simulink model "lqr_quad"  (R2023a)
settings: Solver=VariableStepAuto  StartTime=0.0  StopTime=inf  RelTol=1e-3
undefined symbols (not defined in the file): A_sys, B_sys, C_sys, D_sys
libraries: vrlib x1
settings Model: Creator=sait karadeniz  LastModifiedBy=sait karadeniz
settings DataIOCC: ReturnWorkspaceOutputs=off

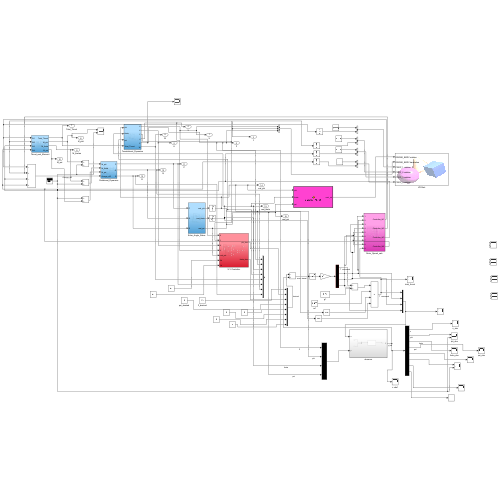
[thumbnail: Simulink's stored preview of the top-level diagram]
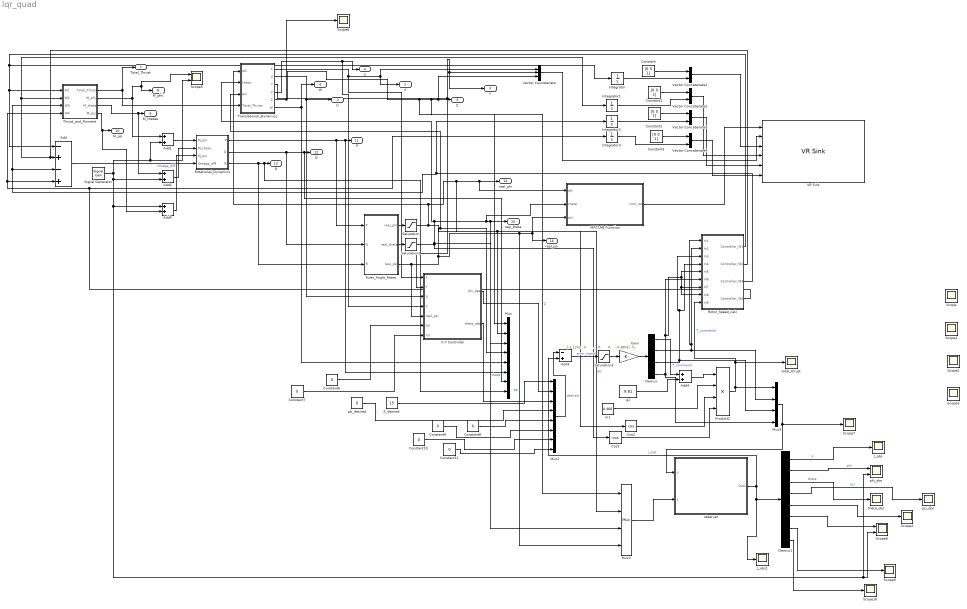
== system lqr_quad ==
  Add : Sum  Inputs=-+-+
  Add{1..2,4..5} (4 alike) : Sum
  Add3 : Sum  Inputs=-+
  Constant{,1..3} (4 alike) : Constant  Value=[0 0 1]  OutMax=[3]
  Constant{6..11} (6 alike) : Constant  Value=0
  Cos2 : Trigonometry  Operator=cos
  Cos3 : Trigonometry  Operator=cos
  Demux : Demux
  Demux1 : Demux  Outputs=8
  Euler_Angle_Rates : Subsystem
  Gain : Gain  Gain=|  Multiplication=Matrix(K*u)
      | [-1.1243,  0,       0,       0,     -0.9940,  0,       0,       0;
      |   0,      -1.6555,  0,       0,      0,      -0.0231,  0,       0;
      |   0,       0,      -2.0992,  0,      0,       0,     -0.1455,  0;
      |   0,       0,       0,     -1.1305,  0,       0,       0,     -0.3803]
  Integrator{,1..3} (4 alike) : Integrator
  MATLAB Function : MATLAB Function  TreatAsAtomicUnit=on
  Mux : Mux  Inputs=8
  Mux1 : Mux  Inputs=8
  Mux2 : Mux
  Mux3 : Mux
  Product2 : Product  Inputs=4
  Rotational_Dynamics : Subsystem
  Rotor_Speed_calc : Subsystem
  Saturation : Saturate  UpperLimit=pi/2  LowerLimit=-pi/2
  Saturation1 : Saturate  UpperLimit=pi/2  LowerLimit=-pi/2
  Saturation3 : Saturate  UpperLimit=500  LowerLimit=-5
  Scope{,1..3,5,8} (6 alike) : Scope  NumInputPorts=2
  Scope{4,6..7,9..10} (5 alike) : Scope
  Signal Generator : SignalGenerator  Amplitude=0.002  Frequency=3  Units=rad/sec
  Thrust_and_Moment : Subsystem
  Translational_Dynamics : Subsystem
  VR Sink : vrlib/VR Sink  InstantiateOnLoad=on  SampleTime=0.1  ViewEnable=on  RemoteChange=off  RemoteView=off  FieldsWritten=DRONE_BODY.rotation.4.1.1.double#DRONE_BODY.translation.3.1.1.double#PROP_1.rotation.4.1.1.double#PROP_2.rotation.4.1.1.double#PROP_3.rotation.4.1.1.double#PROP_4.rotation.4.1.1.double  WorldFileName=C:\Documents\quadcopter.wrl  WorldDescription=Quadcopter World  AutoView=on  VideoDimensions=[]  AllowVariableSize=off  FigureProperties="{'Position', 'Name', 'Viewpoint', 'CameraBound', 'CameraDirection', 'CameraPosition', 'CameraUpVector', 'ZoomFactor', 'Antialiasing', 'Headlight', 'Lighting', 'NavPanel', 'Sound', 'StatusBar', 'Stereo3D', 'Stereo3DCameraOffset', 'Stereo3DHIT', 'ToolBar', 'Textures', 'Transparency', 'Triad', 'Wireframe', 'NavZones', 'NavMode', 'NavSpeed', 'CaptureFileFormat', 'CaptureFileName', 'Record2DCompressMethod', 'Record2DCompressQuality', 'Record2D', 'Record2DFileName', 'Record2DFPS'; [8.8180000000000007e+02   1.8300000000000000e+02   5.7600000000000000e+02   5.0760000000000002e+02], 'Quadcopter World', 'Front View', 'on', [-6.4578595001307049e-01  -1.2433086949529201e-01  -7.5332751287603050e-01], [1.2901758596078691e+01   1.9679088050098620e+01   3.4424497589942021e+01], [-3.6247815328599153e-01  -8.1845083703478472e-01   4.4581141276029251e-01], [1.0000000000000000e+00], 'on', 'on', 'on', 'halfbar', 'on', 'on', 'off', [1.0000000149011612e-01], [0.0000000000000000e+00], 'on', 'on', 'on', 'none', 'off', 'off', 'walk', 'normal', 'tif', '%f_anim_%n.tif', 'auto', [7.5000000000000000e+01], 'off', '%f_anim_%n.avi', 'auto'}"
  Vector Concatenate : Concatenate  NumInputs=3
  Vector Concatenate{1..4} (4 alike) : Concatenate
  X-Y Controller : Subsystem
  Z_desired : Constant  Value=15
  g1 : Constant  Value=9.81
  m1 : Constant  Value=0.468
  observer : Subsystem
  phi_obs : Scope  NumInputPorts=2
  psi_desired : Constant  Value=0
  psi_obs : Scope
  theta_obs : Scope
  total_thrust : Scope
  z_obs : Scope
  z_obs1 : Scope
  X : Outport
  U : Outport  Port=2
  Y : Outport  Port=3
  V : Outport  Port=4
  Z : Outport  Port=5
  W : Outport  Port=6
  Total_Thrust : Outport  Port=7
  M_phii : Outport  Port=8
  M_thetaa : Outport  Port=9
  M_psi : Outport  Port=10
  P : Outport  Port=11
  Q : Outport  Port=12
  R : Outport  Port=13
  real_phi : Outport  Port=14
  real_theta : Outport  Port=15
  real_psi : Outport  Port=16
  wires:
  X-Y Controller/2(theta_des) -> Mux1/3
  Translational_Dynamics/5(Z) -> Scope6/1, Mux2/1, Z/1, Vector Concatenate/3, Mux/1  "Z"
  Z_desired/1 -> Mux1/1
  X-Y Controller/1(phi_des) -> Mux1/2
  Add1/1 -> Rotational_Dynamics/1(M_phi)
  Signal Generator/1 -> Add2/2, Add5/1, phi_obs/2, Scope8/2, Scope5/2, Add1/2
  Integrator3/1 -> Vector Concatenate4/2
  Constant7/1 -> X-Y Controller/7(Yd)
  Euler_Angle_Rates/2(real_theta) -> Saturation1/1
  Constant2/1 -> Vector Concatenate3/1
  Rotor_Speed_calc/1(Controller_W1) -> Add/1, Thrust_and_Moment/1(W1), Integrator/1
  MATLAB Function/1(vrml_rot) -> VR Sink/1
  Rotational_Dynamics/2(Q) -> Euler_Angle_Rates/2(Q), Mux/7, Q/1
  Integrator2/1 -> Vector Concatenate3/2
  Thrust_and_Moment/3(M_theta) -> Add2/1, M_thetaa/1
  Rotor_Speed_calc/2(Controller_W2) -> Integrator1/1, Thrust_and_Moment/2(W2), Add/2
  Translational_Dynamics/1(X) -> Vector Concatenate/1, X/1, X-Y Controller/1(X)
  Vector Concatenate3/1 -> VR Sink/5
  Vector Concatenate2/1 -> VR Sink/4
  Constant3/1 -> Vector Concatenate4/1
  Integrator1/1 -> Vector Concatenate2/2
  Rotor_Speed_calc/4(Controller_W4) -> Thrust_and_Moment/4(W4), Add/4, Integrator3/1
  Vector Concatenate1/1 -> VR Sink/3
  psi_desired/1 -> Mux1/4
  Add/1 -> Rotational_Dynamics/4(Omega_diff)  "Omega_diff"
  Constant1/1 -> Vector Concatenate2/1
  Translational_Dynamics/3(Y) -> Y/1, Vector Concatenate/2, X-Y Controller/2(Y)
  Integrator/1 -> Vector Concatenate1/2
  Vector Concatenate4/1 -> VR Sink/6
  Rotor_Speed_calc/3(Controller_W3) -> Thrust_and_Moment/3(W3), Add/3, Integrator2/1
  Constant6/1 -> X-Y Controller/6(Xd)
  Rotational_Dynamics/3(R) -> Euler_Angle_Rates/3(R), Mux/8, R/1
  Thrust_and_Moment/4(M_psi) -> Add5/2, M_psi/1
  Thrust_and_Moment/2(M_phi) -> M_phii/1, Scope5/1, Add1/1
  Translational_Dynamics/4(V) -> V/1, X-Y Controller/4(V)
  Vector Concatenate/1 -> VR Sink/2
  Translational_Dynamics/6(W) -> W/1, Mux/5
  Translational_Dynamics/2(U) -> U/1, X-Y Controller/3(U)
  Constant/1 -> Vector Concatenate1/1
  Euler_Angle_Rates/1(real_phi) -> Saturation/1
  Thrust_and_Moment/1(Total_Thrust) -> Total_Thrust/1, Translational_Dynamics/4(Total_Thrust)
  Euler_Angle_Rates/3(real_psi) -> Mux/4, Translational_Dynamics/3(psi), Mux2/4, MATLAB Function/3(psi), real_psi/1, X-Y Controller/5(real_psi)  "psi"
  Rotational_Dynamics/1(P) -> Mux/6, P/1, Euler_Angle_Rates/1(P)
  Constant8/1 -> Mux1/5
  Constant9/1 -> Mux1/6
  Constant10/1 -> Mux1/7
  Constant11/1 -> Mux1/8
  Mux1/1 -> Add3/1  "desired"
  Gain/1 -> Demux/1
  Demux/2 -> Mux3/2, Rotor_Speed_calc/1(In1), Rotor_Speed_calc/2(In2)
  Demux/3 -> Rotor_Speed_calc/4(In4), Rotor_Speed_calc/3(In3), Mux3/3
  Demux/4 -> Mux3/4, Rotor_Speed_calc/5(In5), Rotor_Speed_calc/8(In8), Rotor_Speed_calc/7(In7), Rotor_Speed_calc/6(In6)
  Saturation/1 -> Cos2/1, Mux/2, Translational_Dynamics/1(phi), Mux2/2, MATLAB Function/1(phi), real_phi/1  "phi"
  Saturation1/1 -> Cos3/1, Translational_Dynamics/2(theta), Mux2/3, real_theta/1, MATLAB Function/2(theta), Mux/3  "theta"
  g1/1 -> Add4/2
  Cos3/1 -> Product2/4
  m1/1 -> Product2/2
  Product2/1 -> total_thrust/1, Rotor_Speed_calc/9(In9), Mux3/1  "T_command"
  Add4/1 -> Product2/1
  Cos2/1 -> Product2/3
  Demux/1 -> Add4/1  "T_command"
  Add3/1 -> Saturation3/1  "error_signal"
  Saturation3/1 -> Gain/1
  Mux2/1 -> observer/2(y)
  observer/1(Out1) -> Add3/2, z_obs1/1, Demux1/1  "x_hat"
  Demux1/1 -> z_obs/1  "z"
  Demux1/2 -> phi_obs/1  "phi"
  Demux1/3 -> theta_obs/1  "theta"
  Demux1/4 -> psi_obs/1  "psi"
  Mux3/1 -> observer/1(u), Scope7/1
  Demux1/5 -> Scope4/1
  Demux1/6 -> Scope8/1
  Demux1/7 -> Scope9/1
  Demux1/8 -> Scope10/1
  Add2/1 -> Rotational_Dynamics/2(M_theta)
  Add5/1 -> Rotational_Dynamics/3(M_psi)

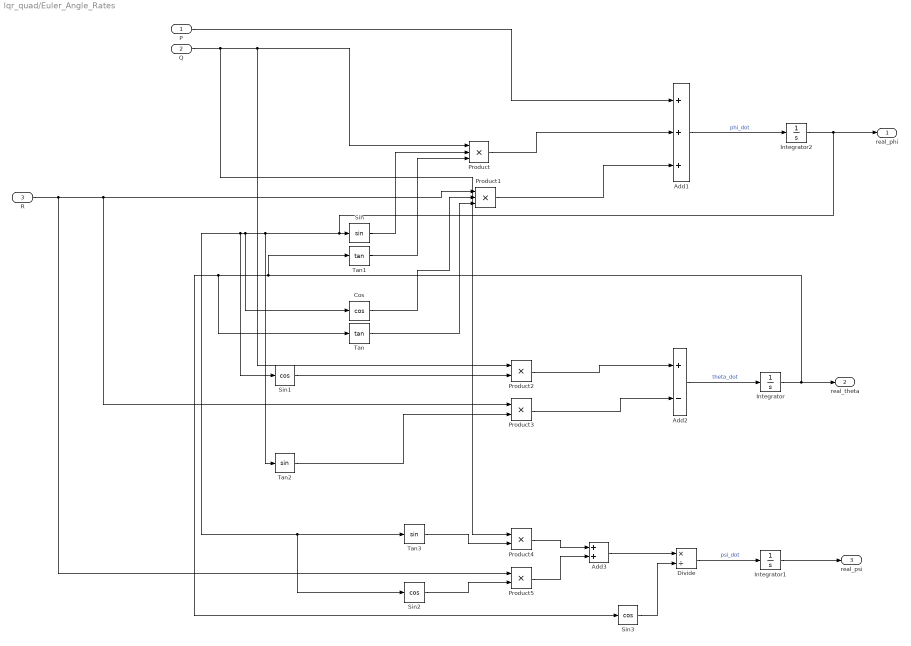
== system lqr_quad/Euler_Angle_Rates ==
  P : Inport
  Q : Inport  Port=2
  R : Inport  Port=3
  Add1 : Sum  Inputs=+++
  Add2 : Sum  Inputs=+-
  Add3 : Sum
  Cos : Trigonometry  Operator=cos
  Divide : Product  Inputs=*/
  Integrator : Integrator
  Integrator1 : Integrator
  Integrator2 : Integrator
  Product : Product  Inputs=3
  Product1 : Product  Inputs=3
  Product{2..5} (4 alike) : Product
  Sin : Trigonometry
  Sin1 : Trigonometry  Operator=cos
  Sin2 : Trigonometry  Operator=cos
  Sin3 : Trigonometry  Operator=cos
  Tan : Trigonometry  Operator=tan
  Tan1 : Trigonometry  Operator=tan
  Tan2 : Trigonometry
  Tan3 : Trigonometry
  real_phi : Outport
  real_theta : Outport  Port=2
  real_psi : Outport  Port=3
  wires:
  Tan1/1 -> Product/3
  Integrator2/1 -> real_phi/1, Sin2/1, Tan3/1, Sin1/1, Cos/1, Tan2/1, Sin/1
  Add1/1 -> Integrator2/1  "phi_dot"
  Divide/1 -> Integrator1/1  "psi_dot"
  Product3/1 -> Add2/2
  Integrator/1 -> real_theta/1, Sin3/1, Tan/1, Tan1/1
  Product1/1 -> Add1/3
  Tan3/1 -> Product4/2
  Sin2/1 -> Product5/2
  Tan2/1 -> Product3/2
  Integrator1/1 -> real_psi/1
  Product2/1 -> Add2/1
  Cos/1 -> Product1/2
  Add2/1 -> Integrator/1  "theta_dot"
  Product4/1 -> Add3/1
  Sin/1 -> Product/2
  Tan/1 -> Product1/3
  Add3/1 -> Divide/1
  Product/1 -> Add1/2
  Sin1/1 -> Product2/2
  Product5/1 -> Add3/2
  Sin3/1 -> Divide/2
  Q/1 -> Product4/1, Product/1, Product2/1
  R/1 -> Product5/1, Product3/1, Product1/1
  P/1 -> Add1/1

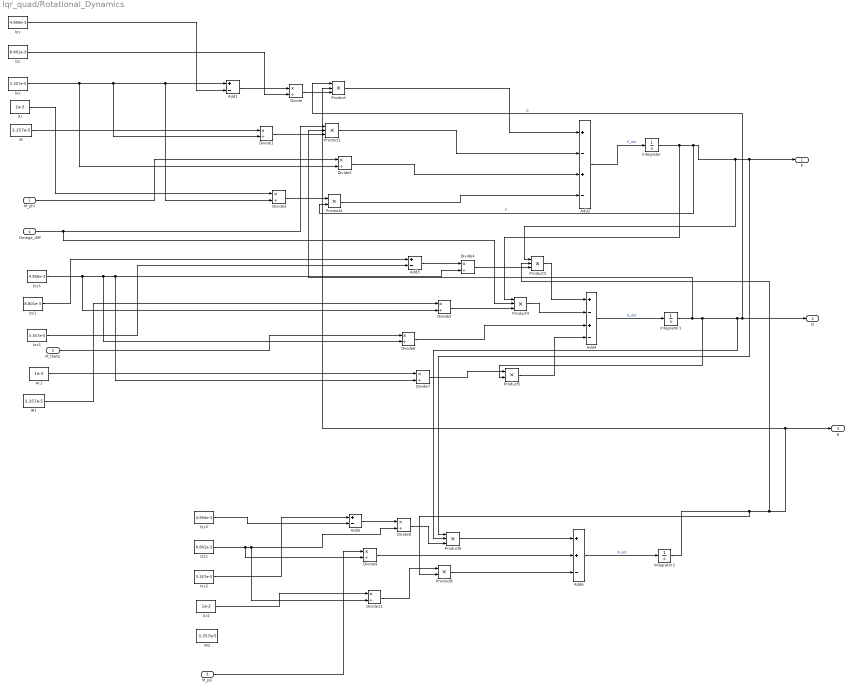
== system lqr_quad/Rotational_Dynamics ==
  M_phi : Inport
  M_theta : Inport  Port=2
  M_psi : Inport  Port=3
  Omega_diff : Inport  Port=4
  Add1 : Sum  Inputs=+-
  Add2 : Sum  Inputs=+-+-
  Add3 : Sum  Inputs=+-
  Add4 : Sum  Inputs=+-+-
  Add5 : Sum  Inputs=+-
  Add6 : Sum  Inputs=++-
  Ar : Constant  Value=1e-3
  Ar1 : Constant  Value=1e-3
  Ar2 : Constant  Value=1e-3
  Divide{,1..9,11} (11 alike) : Product  Inputs=*/
  IR : Constant  Value=3.357e-5
  IR1 : Constant  Value=3.357e-5
  IR2 : Constant  Value=3.357e-5
  Integrator : Integrator
  Integrator1 : Integrator
  Integrator2 : Integrator
  Ixx : Constant  Value=3.357e-5
  Ixx1 : Constant  Value=3.357e-5
  Ixx2 : Constant  Value=3.357e-5
  Iyy : Constant  Value=4.856e-3
  Iyy1 : Constant  Value=4.856e-3
  Iyy2 : Constant  Value=4.856e-3
  Izz : Constant  Value=8.801e-3
  Izz1 : Constant  Value=8.801e-3
  Izz2 : Constant  Value=8.801e-3
  Product{,1,3..4,6} (5 alike) : Product  Inputs=3
  Product2 : Product
  Product5 : Product
  Product8 : Product
  P : Outport
  Q : Outport  Port=2
  R : Outport  Port=3
  wires:
  Integrator/1 -> Product4/1, Product2/2, Product3/1, Product6/1, P/1  "P"
  Product6/1 -> Add6/1
  Add6/1 -> Integrator2/1  "R_dot"
  Divide2/1 -> Add2/3
  Add3/1 -> Divide4/1
  Add5/1 -> Divide8/1
  Divide3/1 -> Product2/1
  Integrator1/1 -> Product1/2, Product5/2, Product/1, Q/1, Product6/2  "Q"
  Product/1 -> Add2/1
  Product1/1 -> Add2/2
  Divide11/1 -> Product8/1
  Add1/1 -> Divide/1
  Product5/1 -> Add4/4
  Integrator2/1 -> Product8/2, Product3/2, R/1, Product/2
  Divide8/1 -> Product6/3
  Product3/1 -> Add4/1
  Add2/1 -> Integrator/1  "P_dot"
  Product2/1 -> Add2/4
  Divide5/1 -> Product4/3
  Divide4/1 -> Product3/3
  Divide6/1 -> Add4/3
  Divide7/1 -> Product5/1
  Product4/1 -> Add4/2
  Add4/1 -> Integrator1/1  "Q_dot"
  Divide9/1 -> Add6/2
  Divide/1 -> Product/3
  Divide1/1 -> Product1/3
  Product8/1 -> Add6/3
  Ixx/1 -> Divide2/2, Divide1/2, Divide3/2, Add1/1
  IR/1 -> Divide1/1
  Omega_diff/1 -> Product4/2, Product1/1
  M_phi/1 -> Divide2/1
  Ar/1 -> Divide3/1
  Iyy/1 -> Add1/2
  Izz/1 -> Divide/2
  Izz1/1 -> Add3/1
  Ixx1/1 -> Add3/2
  Iyy1/1 -> Divide5/2, Divide6/2, Divide7/2, Divide4/2
  IR1/1 -> Divide5/1
  M_theta/1 -> Divide6/1
  Ar1/1 -> Divide7/1
  Ixx2/1 -> Add5/1
  Iyy2/1 -> Add5/2
  Izz2/1 -> Divide9/2, Divide11/2, Divide8/2
  M_psi/1 -> Divide9/1
  Ar2/1 -> Divide11/1

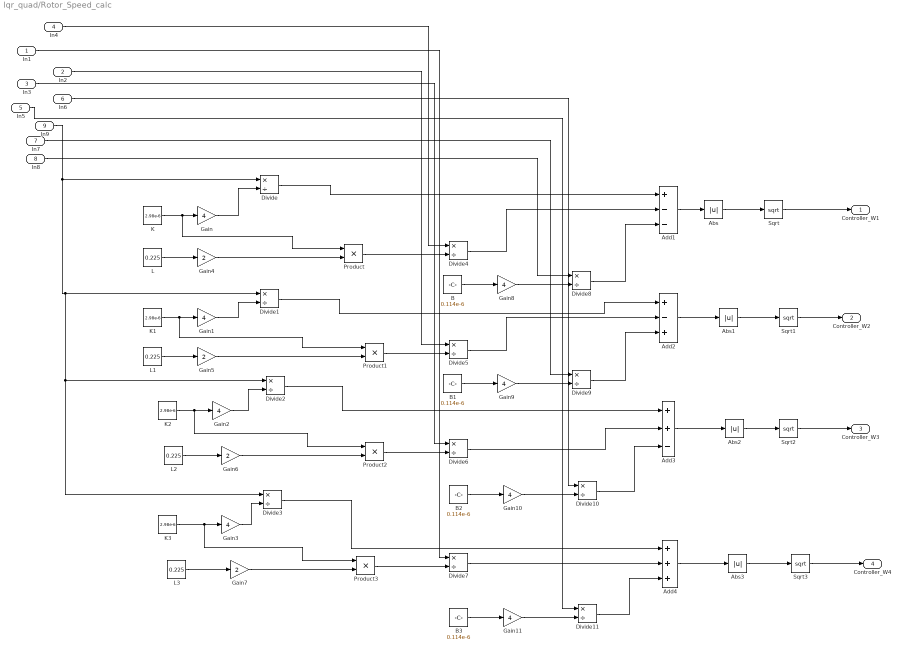
== system lqr_quad/Rotor_Speed_calc ==
  In1 : Inport
  In2 : Inport  Port=2
  In3 : Inport  Port=3
  In4 : Inport  Port=4
  In5 : Inport  Port=5
  In6 : Inport  Port=6
  In7 : Inport  Port=7
  In8 : Inport  Port=8
  In9 : Inport  Port=9
  Abs{,1..3} (4 alike) : Abs  SaturateOnIntegerOverflow=off
  Add1 : Sum  Inputs=+--
  Add2 : Sum  Inputs=+-+
  Add3 : Sum  Inputs=++-
  Add4 : Sum  Inputs=+++
  B{,1..3} (4 alike) : Constant  Value=0.114e-6
  Divide{,1..11} (12 alike) : Product  Inputs=*/
  Gain{,1..3,8..11} (8 alike) : Gain  Gain=4
  Gain{4..7} (4 alike) : Gain  Gain=2
  K{,1..3} (4 alike) : Constant  Value=2.98e-6
  L{,1..3} (4 alike) : Constant  Value=0.225
  Product{,1..3} (4 alike) : Product
  Sqrt{,1..3} (4 alike) : Sqrt
  Controller_W1 : Outport
  Controller_W2 : Outport  Port=2
  Controller_W3 : Outport  Port=3
  Controller_W4 : Outport  Port=4
  wires:
  K/1 -> Product/1, Gain/1
  Sqrt1/1 -> Controller_W2/1
  Divide1/1 -> Add2/1
  Divide/1 -> Add1/1
  Gain3/1 -> Divide3/2
  Gain/1 -> Divide/2
  Divide8/1 -> Add1/3
  Add4/1 -> Abs3/1
  B/1 -> Gain8/1
  B2/1 -> Gain10/1
  Gain5/1 -> Product1/2
  Divide9/1 -> Add2/3
  Abs2/1 -> Sqrt2/1
  Add2/1 -> Abs1/1
  Divide5/1 -> Add2/2
  B3/1 -> Gain11/1
  Add3/1 -> Abs2/1
  Divide11/1 -> Add4/3
  Divide10/1 -> Add3/3
  K1/1 -> Product1/1, Gain1/1
  Divide4/1 -> Add1/2
  In9/1 -> Divide3/1, Divide2/1, Divide1/1, Divide/1
  Product3/1 -> Divide7/2
  Product/1 -> Divide4/2
  K2/1 -> Product2/1, Gain2/1
  Divide2/1 -> Add3/1
  Gain1/1 -> Divide1/2
  Divide3/1 -> Add4/1
  Divide7/1 -> Add4/2
  L1/1 -> Gain5/1
  Gain9/1 -> Divide9/2
  Abs3/1 -> Sqrt3/1
  L/1 -> Gain4/1
  Abs1/1 -> Sqrt1/1
  B1/1 -> Gain9/1
  Sqrt/1 -> Controller_W1/1
  Gain4/1 -> Product/2
  L2/1 -> Gain6/1
  In8/1 -> Divide8/1
  In5/1 -> Divide11/1
  Gain6/1 -> Product2/2
  In3/1 -> Divide6/1
  Product1/1 -> Divide5/2
  Product2/1 -> Divide6/2
  In1/1 -> Divide7/1
  Divide6/1 -> Add3/2
  Gain8/1 -> Divide8/2
  L3/1 -> Gain7/1
  Sqrt3/1 -> Controller_W4/1
  K3/1 -> Product3/1, Gain3/1
  Gain10/1 -> Divide10/2
  Gain7/1 -> Product3/2
  Gain11/1 -> Divide11/2
  Gain2/1 -> Divide2/2
  Sqrt2/1 -> Controller_W3/1
  Abs/1 -> Sqrt/1
  Add1/1 -> Abs/1
  In4/1 -> Divide4/1
  In6/1 -> Divide10/1
  In7/1 -> Divide9/1
  In2/1 -> Divide5/1

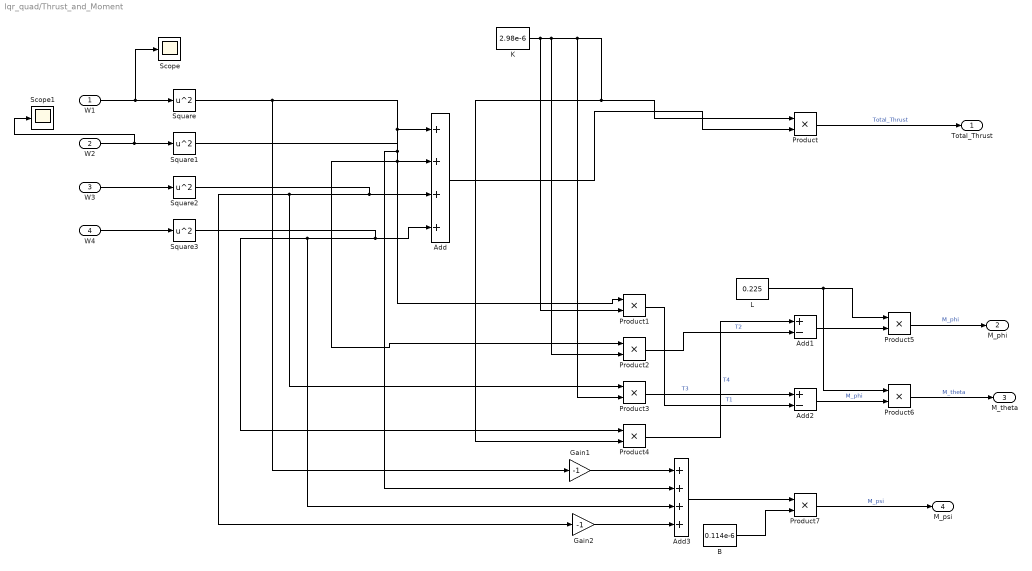
== system lqr_quad/Thrust_and_Moment ==
  W1 : Inport
  W2 : Inport  Port=2
  W3 : Inport  Port=3
  W4 : Inport  Port=4
  Add : Sum  Inputs=++++
  Add1 : Sum  Inputs=+-
  Add2 : Sum  Inputs=+-
  Add3 : Sum  Inputs=++++
  B : Constant  Value=0.114e-6
  Gain1 : Gain  Gain=-1
  Gain2 : Gain  Gain=-1
  K : Constant  Value=2.98e-6
  L : Constant  Value=0.225
  Product{,1..7} (8 alike) : Product
  Scope : Scope
  Scope1 : Scope
  Square{,1..3} (4 alike) : Math  Operator=square
  Total_Thrust : Outport
  M_phi : Outport  Port=2
  M_theta : Outport  Port=3
  M_psi : Outport  Port=4
  wires:
  Square1/1 -> Add3/2, Add/2, Product2/1
  Product3/1 -> Add2/1  "T3"
  Product1/1 -> Add2/2  "T1"
  Square3/1 -> Product4/1, Add3/3, Add/4
  Add3/1 -> Product7/1
  Square2/1 -> Gain2/1, Product3/1, Add/3
  Product7/1 -> M_psi/1  "M_psi"
  W1/1 -> Scope/1, Square/1
  K/1 -> Product2/2, Product4/2, Product/1, Product3/2, Product1/2
  W4/1 -> Square3/1
  Product2/1 -> Add1/2  "T2"
  Add1/1 -> Product5/2
  W2/1 -> Scope1/1, Square1/1
  Product5/1 -> M_phi/1  "M_phi"
  Square/1 -> Add/1, Product1/1, Gain1/1
  Product/1 -> Total_Thrust/1  "Total_Thrust"
  Gain2/1 -> Add3/4
  L/1 -> Product6/1, Product5/1
  Add2/1 -> Product6/2  "M_phi"
  W3/1 -> Square2/1
  B/1 -> Product7/2
  Product4/1 -> Add1/1  "T4"
  Add/1 -> Product/2
  Gain1/1 -> Add3/1
  Product6/1 -> M_theta/1  "M_theta"

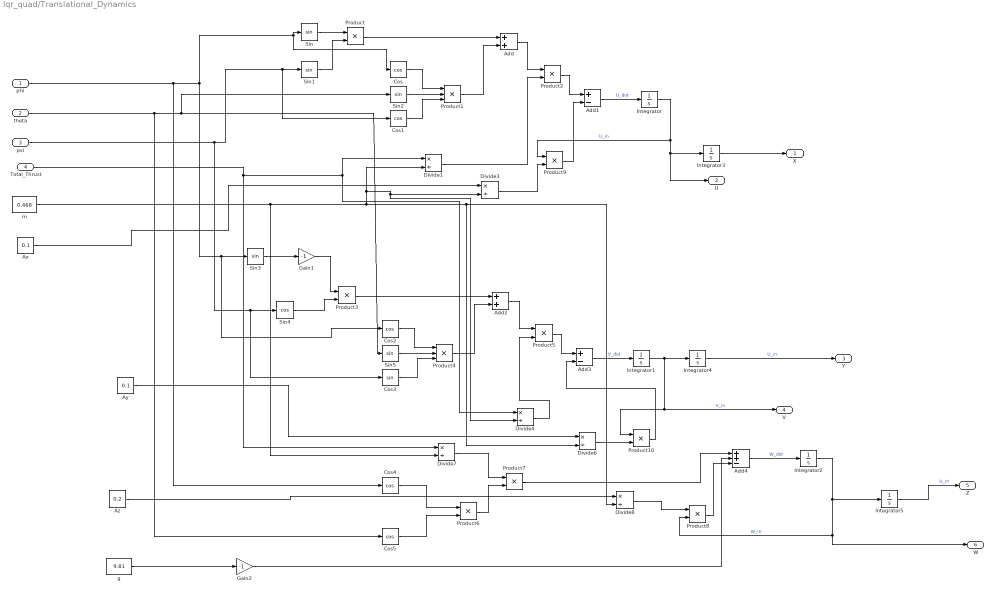
== system lqr_quad/Translational_Dynamics ==
  phi : Inport
  theta : Inport  Port=2
  psi : Inport  Port=3
  Total_Thrust : Inport  Port=4
  Add : Sum
  Add1 : Sum  Inputs=+-
  Add2 : Sum
  Add3 : Sum  Inputs=+-
  Add4 : Sum  Inputs=++-
  Ax : Constant  Value=0.1
  Ay : Constant  Value=0.1
  Az : Constant  Value=0.2
  Cos{,1..2,4..5} (5 alike) : Trigonometry  Operator=cos
  Cos3 : Trigonometry
  Divide{1,3..4,6..8} (6 alike) : Product  Inputs=*/
  Gain1 : Gain  Gain=-1
  Gain2 : Gain  Gain=-1
  Integrator{,1..5} (6 alike) : Integrator
  Product{,2..3,5..10} (9 alike) : Product
  Product1 : Product  Inputs=3
  Product4 : Product  Inputs=3
  Sin{,1..3,5} (5 alike) : Trigonometry
  Sin4 : Trigonometry  Operator=cos
  g : Constant  Value=9.81
  m : Constant  Value=0.468
  X : Outport
  U : Outport  Port=2
  Y : Outport  Port=3
  V : Outport  Port=4
  Z : Outport  Port=5
  W : Outport  Port=6
  wires:
  Integrator1/1 -> Product10/1, V/1, Integrator4/1  "V_in"
  m/1 -> Divide7/2, Divide8/2, Divide6/2, Divide3/2, Divide4/2, Divide1/2
  Integrator2/1 -> Integrator5/1, W/1, Product8/2  "W_in"
  Product8/1 -> Add4/3
  Ay/1 -> Divide6/1
  Product2/1 -> Add1/1
  Integrator/1 -> Product9/1, U/1, Integrator3/1  "U_in"
  g/1 -> Gain2/1
  Product6/1 -> Product7/2
  phi/1 -> Cos2/1, Sin3/1, Sin/1, Cos/1, Cos4/1
  Integrator3/1 -> X/1
  Integrator5/1 -> Z/1  "U_in"
  Product7/1 -> Add4/1
  psi/1 -> Cos3/1, Sin4/1, Cos1/1, Sin1/1
  Product4/1 -> Add2/2
  Divide1/1 -> Product2/2
  Product9/1 -> Add1/2
  Divide7/1 -> Product7/1
  Sin/1 -> Product/1
  theta/1 -> Sin5/1, Sin2/1, Cos5/1
  Gain2/1 -> Add4/2
  Integrator4/1 -> Y/1  "U_in"
  Add/1 -> Product2/1
  Product1/1 -> Add/2
  Cos4/1 -> Product6/1
  Sin2/1 -> Product1/2
  Add1/1 -> Integrator/1  "U_dot"
  Total_Thrust/1 -> Divide7/1, Divide1/1, Divide4/1
  Cos/1 -> Product1/1
  Add3/1 -> Integrator1/1  "V_dot"
  Gain1/1 -> Product3/1
  Sin1/1 -> Product/2
  Add4/1 -> Integrator2/1  "W_dot"
  Cos5/1 -> Product6/2
  Product/1 -> Add/1
  Divide8/1 -> Product8/1
  Az/1 -> Divide8/1
  Divide3/1 -> Product9/2
  Sin5/1 -> Product4/2
  Cos1/1 -> Product1/3
  Ax/1 -> Divide3/1
  Cos3/1 -> Product4/3
  Product10/1 -> Add3/2
  Divide4/1 -> Product5/2
  Add2/1 -> Product5/1
  Sin4/1 -> Product3/2
  Sin3/1 -> Gain1/1
  Divide6/1 -> Product10/2
  Cos2/1 -> Product4/1
  Product3/1 -> Add2/1
  Product5/1 -> Add3/1

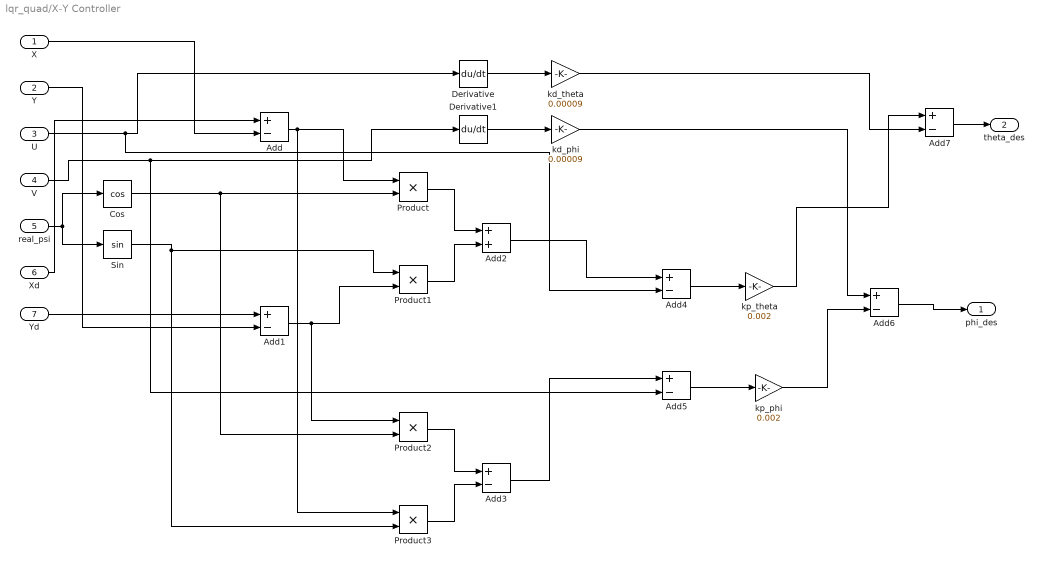
== system lqr_quad/X-Y Controller ==
  X : Inport
  Y : Inport  Port=2
  U : Inport  Port=3
  V : Inport  Port=4
  real_psi : Inport  Port=5
  Xd : Inport  Port=6
  Yd : Inport  Port=7
  Add{,1,3..7} (7 alike) : Sum  Inputs=+-
  Add2 : Sum
  Cos : Trigonometry  Operator=cos
  Derivative : Derivative
  Derivative1 : Derivative
  Product{,1..3} (4 alike) : Product
  Sin : Trigonometry
  kd_phi : Gain  Gain=0.00009
  kd_theta : Gain  Gain=0.00009
  kp_phi : Gain  Gain=0.002
  kp_theta : Gain  Gain=0.002
  phi_des : Outport
  theta_des : Outport  Port=2
  wires:
  X/1 -> Add/2
  Xd/1 -> Add/1
  Yd/1 -> Add1/1
  Y/1 -> Add1/2
  real_psi/1 -> Sin/1, Cos/1
  Cos/1 -> Product2/2, Product/2
  Add/1 -> Product3/1, Product/1
  Add1/1 -> Product2/1, Product1/2
  Sin/1 -> Product1/1, Product3/2
  Product1/1 -> Add2/2
  Product/1 -> Add2/1
  Add2/1 -> Add4/1
  Product2/1 -> Add3/1
  Product3/1 -> Add3/2
  Add3/1 -> Add5/1
  U/1 -> Add4/2, Derivative/1
  V/1 -> Add5/2, Derivative1/1
  Derivative/1 -> kd_theta/1
  Derivative1/1 -> kd_phi/1
  Add4/1 -> kp_theta/1
  Add5/1 -> kp_phi/1
  kd_phi/1 -> Add6/1
  kp_phi/1 -> Add6/2
  kp_theta/1 -> Add7/1
  kd_theta/1 -> Add7/2
  Add6/1 -> phi_des/1
  Add7/1 -> theta_des/1

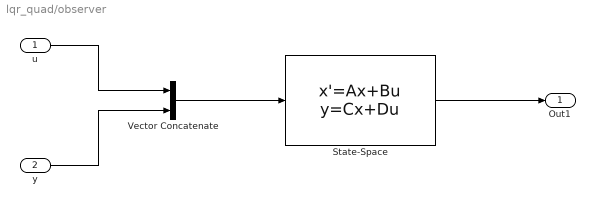
== system lqr_quad/observer ==
  u : Inport
  y : Inport  Port=2
  State-Space : StateSpace  A=A_sys  B=B_sys  C=C_sys  D=D_sys  InitialCondition=zeros(8,1)
  Vector Concatenate : Concatenate
  Out1 : Outport
  wires:
  u/1 -> Vector Concatenate/1
  y/1 -> Vector Concatenate/2
  Vector Concatenate/1 -> State-Space/1
  State-Space/1 -> Out1/1

== matlab function lqr_quad/MATLAB Function ==
  data: phi input; vrml_rot output; theta input; psi input
function vrml_rot = EulerToVRMLRot(phi, theta, psi)
% Bu fonksiyon, roll (phi), pitch (theta) ve yaw (psi) Euler açılarını
% VRML'nin beklediği Axis-Angle formatına dönüştürür.
% Girişler (radyan cinsinden):
% phi   : Roll açısı (X ekseni etrafında)
% theta : Pitch açısı (Y ekseni etrafında)
% psi   : Yaw açısı (Z ekseni etrafında)
% Çıkış (Axis-Angle formatında):
% vrml_rot = [eksen_x, eksen_y, eksen_z, açı_radyan]

% Genellikle MATLAB ve VRML arasındaki koordinat sistemi farklarını
% ve Euler açı sıra konvansiyonunu dikkate almak gerekir.
% Burada Z-Y-X (Yaw-Pitch-Roll) Euler dönüşüm sırasını kullanarak bir
% dönüşüm matrisi oluşturup, ardından bu matristen Axis-Angle'a dönüştüreceğiz.
% Simulink'teki VRML Viewer genellikle Z-Y-X konvansiyonunu iyi karşılar.

% Dönüşüm Matrisi Oluşturma (Z-Y-X Euler açısı sırası)
% R = Rz(psi) * Ry(theta) * Rx(phi)
Rx = [1 0 0; 0 cos(phi) -sin(phi); 0 sin(phi) cos(phi)];
Ry = [cos(theta) 0 sin(theta); 0 1 0; -sin(theta) 0 cos(theta)];
Rz = [cos(psi) -sin(psi) 0; sin(psi) cos(psi) 0; 0 0 1];

RotationMatrix = Rz * Ry * Rx;

% Dönüşüm Matrisinden Axis-Angle'a Dönüştürme
% (Bu dönüşüm için temel bir algoritma kullanılmıştır)
traceR = RotationMatrix(1,1) + RotationMatrix(2,2) + RotationMatrix(3,3);
angle = acos((traceR - 1) / 2);

if abs(angle) < 1e-6 % Açı çok küçükse veya sıfırsa
    axis = [0 0 1]; % Herhangi bir eksen olabilir, Z varsayalım
    angle = 0;
elseif abs(angle - pi) < 1e-6 % Açı 180 derece ise
    % Bu durum için daha dikkatli hesaplama gerekir,
    % örneğin sütunlar arası farklardan eksen bulunur.
    % Şimdilik bu durumu basitleştirelim veya varsayalım ki nadir olacak.
    % Daha sağlam bir yaklaşım için https://www.euclideanspace.com/maths/geometry/rotations/conversions/matrixToAngle/index.htm
    % gibi kaynaklara başvurulabilir.
    % Basit bir 180 derece dönüş ekseni bulma:
    axis_x = RotationMatrix(1,1) + 1;
    axis_y = RotationMatrix(2,2) + 1;
    axis_z = RotationMatrix(3,3) + 1;
    % En büyük bileşeni bulup normalize et
    max_val = max([axis_x, axis_y, axis_z]);
    if max_val == 0
        axis = [1 0 0]; % Varsayılan
    else
        axis = [axis_x, axis_y, axis_z] / max_val; % Normalizasyon sadece yönü korur.
    end
else
    % Normal durum
    axis_x = RotationMatrix(3,2) - RotationMatrix(2,3);
    axis_y = RotationMatrix(1,3) - RotationMatrix(3,1);
    axis_z = RotationMatrix(2,1) - RotationMatrix(1,2);
    axis_magnitude = norm([axis_x, axis_y, axis_z]);

    if axis_magnitude < 1e-6 % Neredeyse sıfır dönme
        axis = [0 0 1]; % Varsayılan
        angle = 0;
    else
        axis = [axis_x, axis_y, axis_z] / axis_magnitude;
    end
end

vrml_rot = [axis(1); axis(2); axis(3); angle];

end
